simulink model "Sim_excitedBLWN"  (R2016b)
settings: Solver=FixedStepAuto  StartTime=0.0  StopTime=Tsim  FixedStep=dtint  RelTol=1e-3
values from neighbouring files (symbols this model uses):
  As = [zeros(3,3),eye(3,3) ... (first row only)    [StructModel_BLWN.m]
  Bs = [zeros(3,1) ... (first row only)    [StructModel_BLWN.m]
  Cs = [eye(DoF)+diag(-ones(DoF-1,1),-1),zeros(DoF)]    [StructModel_BLWN.m]
  Ds = zeros(DoF,1)    [StructModel_BLWN.m]
settings Model: Creator=dsmj  LastModifiedBy=dsmj

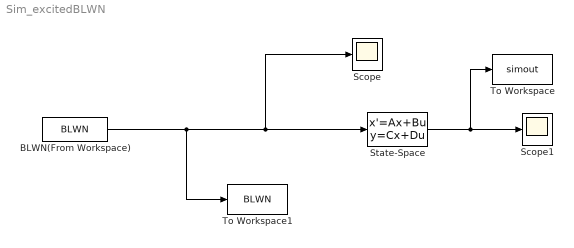
== system Sim_excitedBLWN ==
  BLWN(From Workspace) : FromWorkspace  VariableName=BLWN  SampleTime=0
  Scope : Scope
  Scope1 : Scope
  State-Space : StateSpace  A=As  B=Bs  C=Cs  D=Ds  X0=0
  To Workspace : ToWorkspace  VariableName=simout  SaveFormat=Timeseries  SampleTime=-1
  To Workspace1 : ToWorkspace  VariableName=BLWN  SaveFormat=Timeseries  SampleTime=-1
  wires:
  State-Space/1 -> To Workspace/1, Scope1/1
  BLWN(From Workspace)/1 -> To Workspace1/1, Scope/1, State-Space/1
